simulink model "testDrydenSimulink"  (R2021a)
settings: Solver=VariableStepAuto  StartTime=0.0  StopTime=10.0  RelTol=1e-3
values from neighbouring files (symbols this model uses):
  F = [0;0;0]    [simple_sim.m]
  q = uKF(2)    [dynJacobian.m]    (also in getDynamicsJacobian.m; getDynamicsJacobianTest.m; getStateTransitionDynamics.m; simple_sim.m)
  r = uKF(3)    [dynJacobian.m]    (also in getDynamicsJacobian.m; getDynamicsJacobianTest.m; getStateTransitionDynamics.m; simple_sim.m)
undefined symbols (not defined in the file or in its folder): Light, MIL
libraries: aerolibtransform2 x1, aerolibwind2 x1
settings Model: Creator=vishnu.vithala  LastModifiedBy=vishnu.vithala

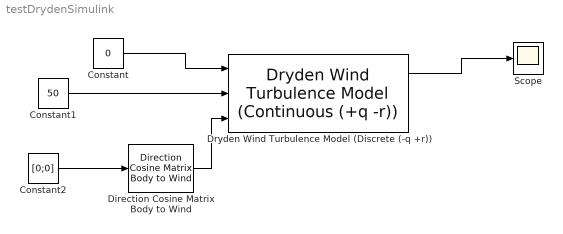
== system testDrydenSimulink ==
  Constant : Constant  Value=0
  Constant1 : Constant  Value=50
  Constant2 : Constant  Value=[0;0]
  Direction Cosine Matrix Body to Wind : aerolibtransform2/Direction Cosine Matrix Body to Wind
      settings: SourceProductBaseCode=AE
  Dryden Wind Turbulence Model (Discrete (-q +r)) : aerolibwind2/Dryden Wind Turbulence Model  (Continuous (+q -r))  units=Metric (MKS)  spec=MIL-F-8785C  model=Discrete Dryden (-q +r)  W20=15  Wdeg=0  TurbProb=10^-2 - Light  L_high=533.4  Wingspan=10  ts=0.1  Seed=[23341 23342 23343 23344]  T_on=on
  Scope : Scope
  wires:
  Constant/1 -> Dryden Wind Turbulence Model (Discrete (-q +r))/1
  Constant1/1 -> Dryden Wind Turbulence Model (Discrete (-q +r))/2
  Dryden Wind Turbulence Model (Discrete (-q +r))/1 -> Scope/1
  Constant2/1 -> Direction Cosine Matrix Body to Wind/1
  Direction Cosine Matrix Body to Wind/1 -> Dryden Wind Turbulence Model (Discrete (-q +r))/3
